simulink model "roboterrestreESC2014aslx_PRINT"  (R2015a)
settings: Solver=ode1  StartTime=0.0  StopTime=Tsimu  FixedStep=passo  RelTol=1e-3
undefined symbols (not defined in the file or in its folder): h, Kesc, N, x0
settings Model: CovModelRefEnable=off  Creator=alessandropeixoto  LastModifiedBy=Jean
settings DataIOCC: SaveFormat=StructureWithTime
settings HardwareCC: ProdBitPerPointer=64  ProdLargestAtomicFloat=Float  ProdIntDivRoundTo=Zero  ProdEndianess=LittleEndian  ProdHWDeviceType=Specified
settings GRTTargetCC: GeneratePreprocessorConditionals=Use local settings

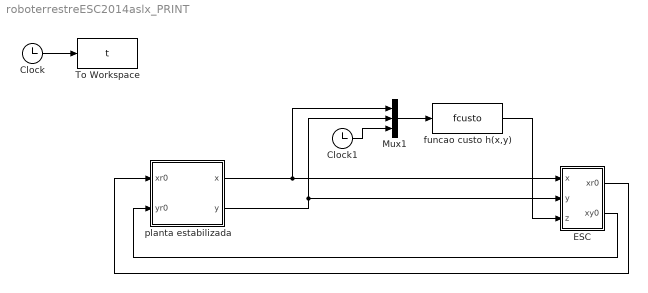
== system roboterrestreESC2014aslx_PRINT ==
  Clock : Clock
  Clock1 : Clock
  ESC : Subsystem
  Mux1 : Mux  Inputs=3
  To Workspace : ToWorkspace  VariableName=t  SampleTime=-1
  funcao custo h(x,y) : MATLABFcn  MATLABFcn=fcusto
  planta estabilizada : Subsystem
  wires:
  planta estabilizada/1(x) -> ESC/1(x), Mux1/1
  planta estabilizada/2(y) -> Mux1/2, ESC/2(y)
  Clock/1 -> To Workspace/1
  Clock1/1 -> Mux1/3
  Mux1/1 -> funcao custo h(x,y)/1
  ESC/2(xy0) -> planta estabilizada/2(yr0)
  ESC/1(xr0) -> planta estabilizada/1(xr0)
  funcao custo h(x,y)/1 -> ESC/3(z)

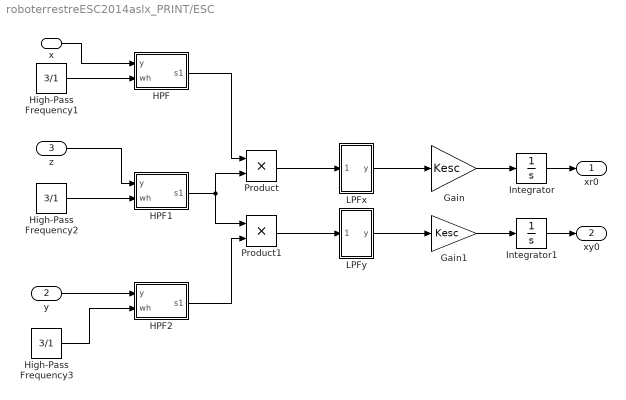
== system roboterrestreESC2014aslx_PRINT/ESC ==
  x : Inport
  y : Inport  Port=2
  z : Inport  Port=3
  Gain : Gain  Gain=Kesc
  Gain1 : Gain  Gain=Kesc
  HPF : Subsystem
  HPF1 : Subsystem
  HPF2 : Subsystem
  High-Pass Frequency1 : Constant  Value=3/1  SampleTime=Inf
  High-Pass Frequency2 : Constant  Value=3/1  SampleTime=Inf
  High-Pass Frequency3 : Constant  Value=3/1  SampleTime=Inf
  Integrator : Integrator  InitialCondition=1
  Integrator1 : Integrator  InitialCondition=1
  LPFx : Subsystem
  LPFy : Subsystem
  Product : Product
  Product1 : Product
  xr0 : Outport
  xy0 : Outport  Port=2
  wires:
  HPF2/1(s1) -> Product1/2
  Gain/1 -> Integrator/1
  LPFy/1(y) -> Gain1/1
  x/1 -> HPF/1(y)
  Integrator1/1 -> xy0/1
  Integrator/1 -> xr0/1
  HPF/1(s1) -> Product/1
  Product1/1 -> LPFy/1(In1)
  HPF1/1(s1) -> Product1/1, Product/2
  Product/1 -> LPFx/1(In1)
  LPFx/1(y) -> Gain/1
  High-Pass Frequency1/1 -> HPF/2(wh)
  z/1 -> HPF1/1(y)
  High-Pass Frequency2/1 -> HPF1/2(wh)
  y/1 -> HPF2/1(y)
  High-Pass Frequency3/1 -> HPF2/2(wh)
  Gain1/1 -> Integrator1/1

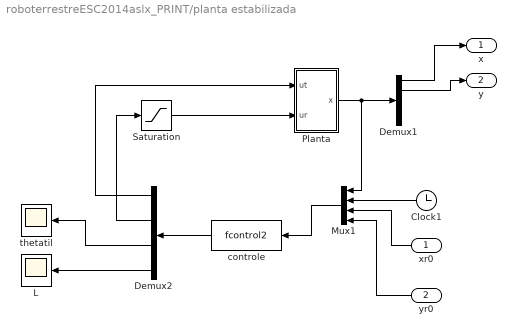
== system roboterrestreESC2014aslx_PRINT/planta estabilizada ==
  xr0 : Inport
  yr0 : Inport  Port=2
  Clock1 : Clock
  Demux1 : Demux  Outputs=5
  Demux2 : Demux
  L : Scope
      settings: YMin=-0.16559  YMax=1.54394  SaveName=ScopeData6
  Mux1 : Mux
  Planta : Subsystem
  Saturation : Saturate  UpperLimit=10  LowerLimit=-10
  controle : MATLABFcn  MATLABFcn=fcontrol2
  thetatil : Scope
      settings: YMin=-7370.79779  YMax=59109.94409  SaveName=ScopeData5
  x : Outport
  y : Outport  Port=2
  wires:
  controle/1 -> Demux2/1
  Planta/1(x) -> Demux1/1, Mux1/1
  Clock1/1 -> Mux1/2
  Demux2/2 -> Saturation/1
  yr0/1 -> Mux1/4
  Demux2/4 -> L/1
  Mux1/1 -> controle/1
  Demux2/3 -> thetatil/1
  Demux2/1 -> Planta/1(ut)
  xr0/1 -> Mux1/3
  Demux1/1 -> x/1
  Demux1/2 -> y/1
  Saturation/1 -> Planta/2(ur)

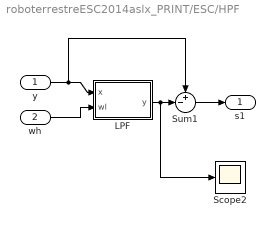
== system roboterrestreESC2014aslx_PRINT/ESC/HPF ==
  y : Inport
  wh : Inport  Port=2
  LPF : Subsystem
  Scope2 : Scope
      settings: YMin=0.6  YMax=1.125  SaveName=ScopeData5
  Sum1 : Sum  Inputs=+-|
  s1 : Outport
  wires:
  LPF/1(y) -> Sum1/2, Scope2/1
  wh/1 -> LPF/2(wl)
  Sum1/1 -> s1/1
  y/1 -> Sum1/1, LPF/1(x)

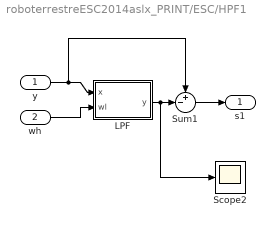
== system roboterrestreESC2014aslx_PRINT/ESC/HPF1 ==
  y : Inport
  wh : Inport  Port=2
  LPF : Subsystem
  Scope2 : Scope
      settings: YMin=0.6  YMax=1.125  SaveName=ScopeData5
  Sum1 : Sum  Inputs=+-|
  s1 : Outport
  wires:
  y/1 -> LPF/1(x), Sum1/1
  Sum1/1 -> s1/1
  wh/1 -> LPF/2(wl)
  LPF/1(y) -> Scope2/1, Sum1/2

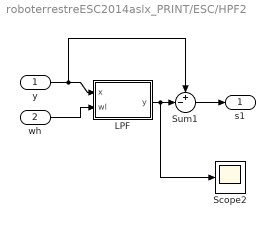
== system roboterrestreESC2014aslx_PRINT/ESC/HPF2 ==
  y : Inport
  wh : Inport  Port=2
  LPF : Subsystem
  Scope2 : Scope
      settings: YMin=0.6  YMax=1.125  SaveName=ScopeData5
  Sum1 : Sum  Inputs=+-|
  s1 : Outport
  wires:
  y/1 -> LPF/1(x), Sum1/1
  Sum1/1 -> s1/1
  wh/1 -> LPF/2(wl)
  LPF/1(y) -> Scope2/1, Sum1/2

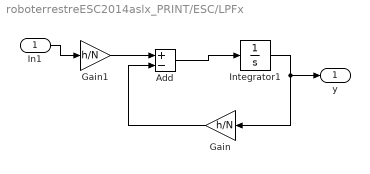
== system roboterrestreESC2014aslx_PRINT/ESC/LPFx ==
  In1 : Inport
  Add : Sum  Inputs=+-
  Gain : Gain  Gain=h/N
  Gain1 : Gain  Gain=h/N
  Integrator1 : Integrator
  y : Outport
  wires:
  Add/1 -> Integrator1/1
  In1/1 -> Gain1/1
  Gain/1 -> Add/2
  Integrator1/1 -> y/1, Gain/1
  Gain1/1 -> Add/1

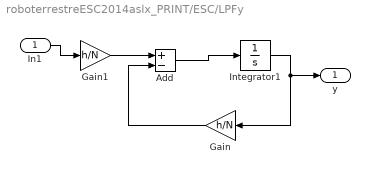
== system roboterrestreESC2014aslx_PRINT/ESC/LPFy ==
  In1 : Inport
  Add : Sum  Inputs=+-
  Gain : Gain  Gain=h/N
  Gain1 : Gain  Gain=h/N
  Integrator1 : Integrator
  y : Outport
  wires:
  Add/1 -> Integrator1/1
  In1/1 -> Gain1/1
  Gain/1 -> Add/2
  Integrator1/1 -> y/1, Gain/1
  Gain1/1 -> Add/1

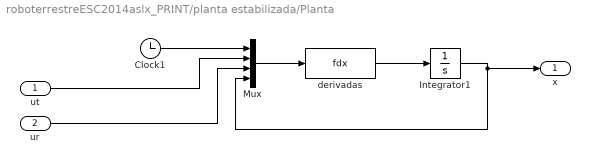
== system roboterrestreESC2014aslx_PRINT/planta estabilizada/Planta ==
  ut : Inport
  ur : Inport  Port=2
  Clock1 : Clock
  Integrator1 : Integrator  InitialCondition=x0
  Mux : Mux
  derivadas : MATLABFcn  MATLABFcn=fdx
  x : Outport
  wires:
  ur/1 -> Mux/3
  ut/1 -> Mux/2
  Clock1/1 -> Mux/1
  Mux/1 -> derivadas/1
  Integrator1/1 -> x/1, Mux/4
  derivadas/1 -> Integrator1/1

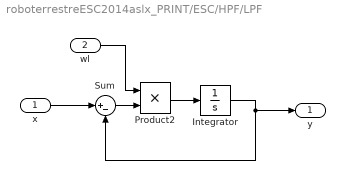
== system roboterrestreESC2014aslx_PRINT/ESC/HPF/LPF ==
  x : Inport
  wl : Inport  Port=2
  Integrator : Integrator
  Product2 : Product
  Sum : Sum  Inputs=|+-
  y : Outport
  wires:
  wl/1 -> Product2/1
  Integrator/1 -> y/1, Sum/2
  Product2/1 -> Integrator/1
  Sum/1 -> Product2/2
  x/1 -> Sum/1

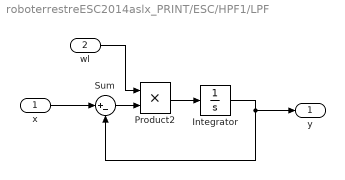
== system roboterrestreESC2014aslx_PRINT/ESC/HPF1/LPF ==
  x : Inport
  wl : Inport  Port=2
  Integrator : Integrator
  Product2 : Product
  Sum : Sum  Inputs=|+-
  y : Outport
  wires:
  x/1 -> Sum/1
  Sum/1 -> Product2/2
  Product2/1 -> Integrator/1
  Integrator/1 -> Sum/2, y/1
  wl/1 -> Product2/1

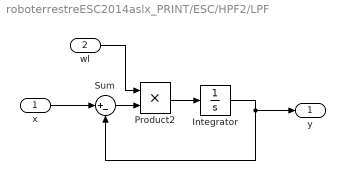
== system roboterrestreESC2014aslx_PRINT/ESC/HPF2/LPF ==
  x : Inport
  wl : Inport  Port=2
  Integrator : Integrator
  Product2 : Product
  Sum : Sum  Inputs=|+-
  y : Outport
  wires:
  x/1 -> Sum/1
  Sum/1 -> Product2/2
  Product2/1 -> Integrator/1
  Integrator/1 -> Sum/2, y/1
  wl/1 -> Product2/1
